simulink model "conf_paper_trajectory"  (R2023a)
settings: Solver=VariableStepAuto  StartTime=0.0  StopTime=75  RelTol=1e-3
undefined symbols (not defined in the file): Aircraft
libraries: simulink x2
settings Model: Creator=abhandari1  LastModifiedBy=abhandari1

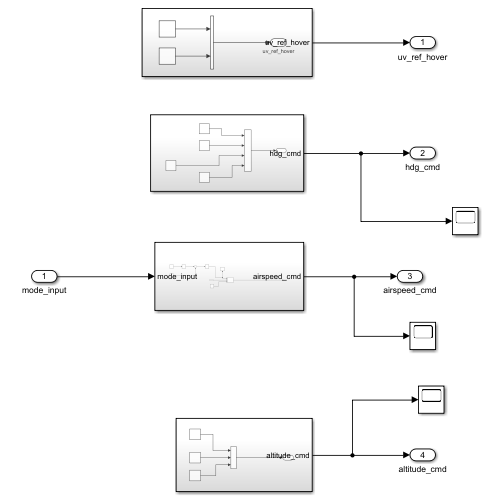
[thumbnail: Simulink's stored preview of the top-level diagram]
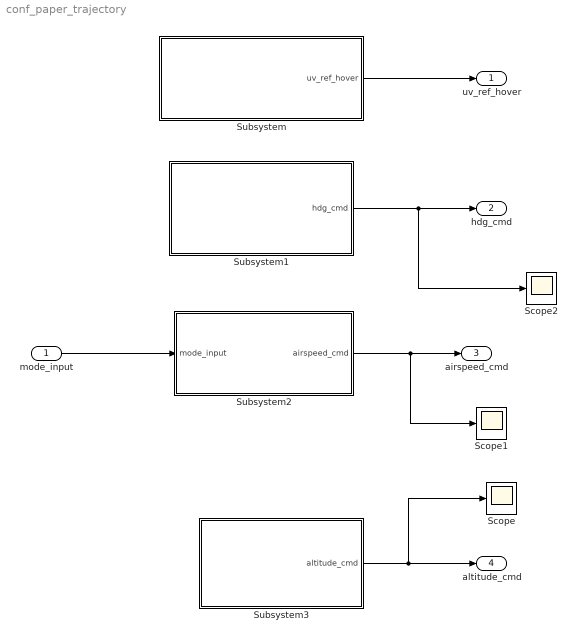
== system conf_paper_trajectory ==
  mode_input : Inport
  Scope : Scope
  Scope1 : Scope
  Scope2 : Scope
  Subsystem : Subsystem
  Subsystem1 : Subsystem
  Subsystem2 : Subsystem
  Subsystem3 : Subsystem
  uv_ref_hover : Outport
  hdg_cmd : Outport  Port=2
  airspeed_cmd : Outport  Port=3
  altitude_cmd : Outport  Port=4
  wires:
  Subsystem1/1(hdg_cmd) -> Scope2/1, hdg_cmd/1
  Subsystem2/1(airspeed_cmd) -> Scope1/1, airspeed_cmd/1
  mode_input/1 -> Subsystem2/1(mode_input)
  Subsystem3/1(altitude_cmd) -> Scope/1, altitude_cmd/1
  Subsystem/1(uv_ref_hover) -> uv_ref_hover/1

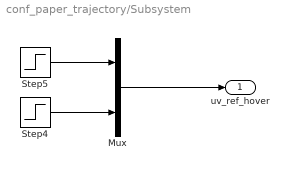
== system conf_paper_trajectory/Subsystem ==
  Mux : Mux  Inputs=2
  Step4 : Step  Time=73  After=3  OutDataTypeStr=single  SampleTime=0
  Step5 : Step  Time=27  After=0  OutDataTypeStr=single  SampleTime=0
  uv_ref_hover : Outport
  wires:
  Step5/1 -> Mux/1
  Mux/1 -> uv_ref_hover/1
  Step4/1 -> Mux/2

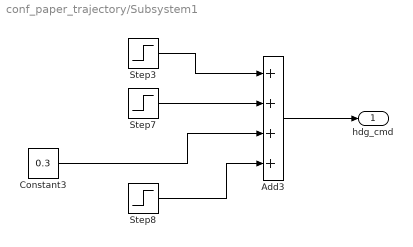
== system conf_paper_trajectory/Subsystem1 ==
  Add3 : Sum  Inputs=++++
  Constant3 : Constant  Value=0.3  OutDataTypeStr=single
  Step3 : Step  Time=2  After=-0.8  OutDataTypeStr=single  SampleTime=0
  Step7 : Step  Time=14  Before=-0.8  After=0.5  OutDataTypeStr=single  SampleTime=0
  Step8 : Step  Time=25  Before=0.5  After=2.75  OutDataTypeStr=single  SampleTime=0
  hdg_cmd : Outport
  wires:
  Step7/1 -> Add3/2
  Step8/1 -> Add3/4
  Constant3/1 -> Add3/3
  Add3/1 -> hdg_cmd/1
  Step3/1 -> Add3/1

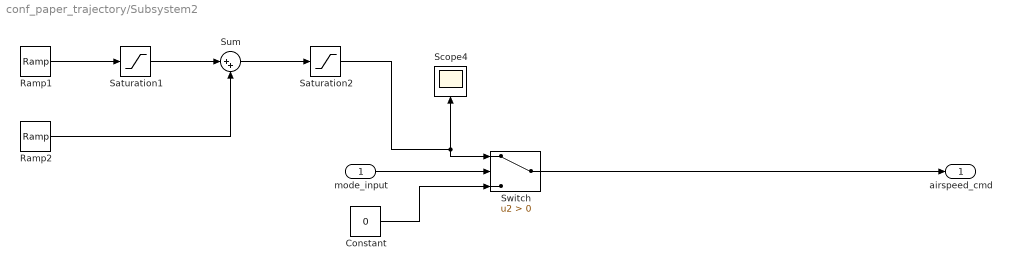
== system conf_paper_trajectory/Subsystem2 ==
  mode_input : Inport
  Constant : Constant  Value=0  OutDataTypeStr=single
  Ramp1 : simulink/Sources/Ramp  slope=Aircraft.Control.modes.hover2forward_airspeed_ramp  start=7  InitialOutput=0
  Ramp2 : simulink/Sources/Ramp  slope=Aircraft.Control.modes.forward2hover_airspeed_ramp  start=52  InitialOutput=0
  Saturation1 : Saturate  UpperLimit=22  LowerLimit=0  OutDataTypeStr=single
  Saturation2 : Saturate  UpperLimit=22  LowerLimit=0  OutDataTypeStr=single
  Scope4 : Scope
  Sum : Sum  Inputs=|++
  Switch : Switch  Criteria=u2 > Threshold  SaturateOnIntegerOverflow=off  InputSameDT=off
  airspeed_cmd : Outport
  wires:
  Ramp1/1 -> Saturation1/1
  Constant/1 -> Switch/3
  Ramp2/1 -> Sum/2
  Saturation2/1 -> Switch/1, Scope4/1
  Sum/1 -> Saturation2/1
  Saturation1/1 -> Sum/1
  mode_input/1 -> Switch/2
  Switch/1 -> airspeed_cmd/1

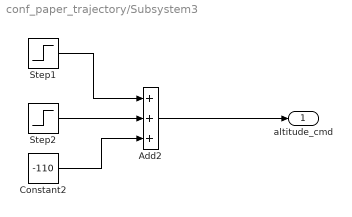
== system conf_paper_trajectory/Subsystem3 ==
  Add2 : Sum  Inputs=+++
  Constant2 : Constant  Value=-110  OutDataTypeStr=single
  Step1 : Step  Time=15  Before=100  After=110  OutDataTypeStr=single  SampleTime=0
  Step2 : Step  Time=40  Before=110  After=90  OutDataTypeStr=single  SampleTime=0
  altitude_cmd : Outport
  wires:
  Add2/1 -> altitude_cmd/1
  Step2/1 -> Add2/2
  Constant2/1 -> Add2/3
  Step1/1 -> Add2/1
